simulink model "inclass0912"  (R2022b)
settings: Solver=VariableStepAuto  StartTime=0.0  StopTime=20.0  RelTol=1e-3
settings Model: Creator=sprinkle  LastModifiedBy=sprinkle

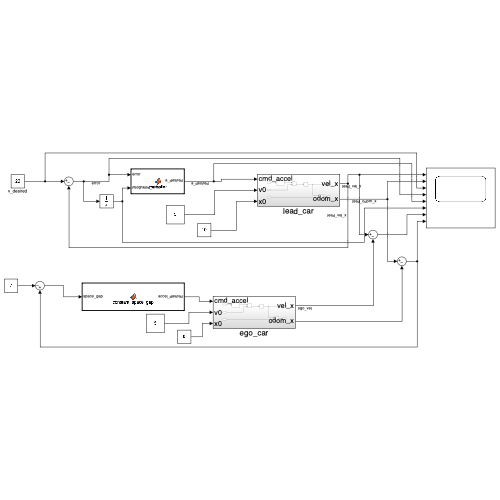
[thumbnail: Simulink's stored preview of the top-level diagram]
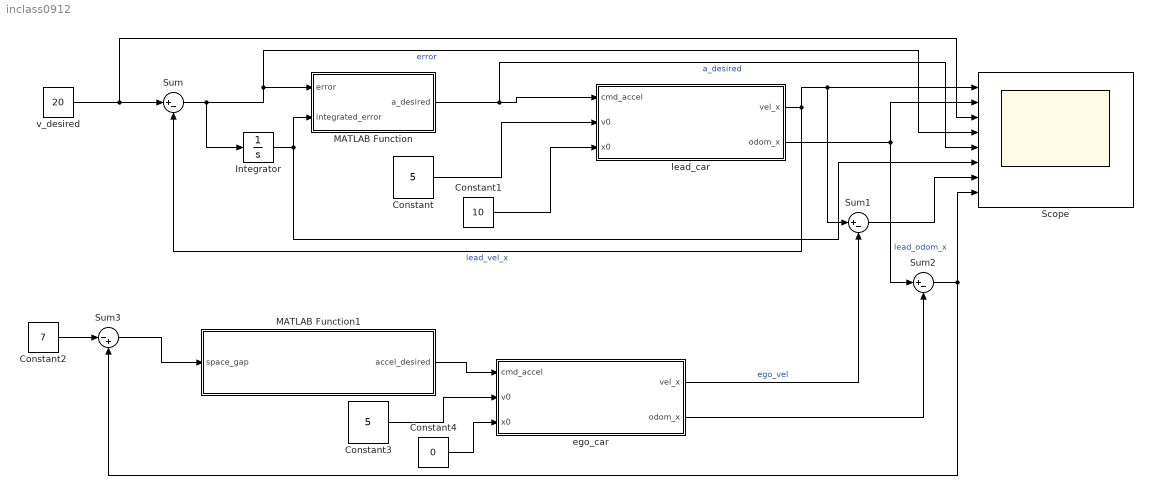
== system inclass0912 ==
  Constant : Constant  Value=5
  Constant1 : Constant  Value=10
  Constant2 : Constant  Value=7
  Constant3 : Constant  Value=5
  Constant4 : Constant  Value=0
  Integrator : Integrator
  MATLAB Function : MATLAB Function  TreatAsAtomicUnit=on
  MATLAB Function1 : MATLAB Function  TreatAsAtomicUnit=on
  Scope : Scope  NumInputPorts=8
  Sum : Sum  Inputs=|+-
  Sum1 : Sum  Inputs=|+-
  Sum2 : Sum  Inputs=|+-
  Sum3 : Sum  Inputs=|-+
  ego_car : Subsystem
  lead_car : Subsystem
  v_desired : Constant  Value=20
  wires:
  Constant/1 -> lead_car/2(v0)
  Constant1/1 -> lead_car/3(x0)
  MATLAB Function/1(a_desired) -> Scope/5, lead_car/1(cmd_accel)  "a_desired"
  lead_car/1(vel_x) -> Sum1/1, Scope/1, Sum/2  "lead_vel_x"
  lead_car/2(odom_x) -> Sum2/1, Scope/2  "lead_odom_x"
  v_desired/1 -> Scope/3, Sum/1
  Sum/1 -> Integrator/1, Scope/4, MATLAB Function/1(error)  "error"
  Integrator/1 -> Scope/6, MATLAB Function/2(integrated_error)
  ego_car/1(vel_x) -> Sum1/2  "ego_vel"
  ego_car/2(odom_x) -> Sum2/2
  Constant2/1 -> Sum3/1
  Sum2/1 -> Scope/8, Sum3/2
  Sum3/1 -> MATLAB Function1/1(space_gap)
  MATLAB Function1/1(accel_desired) -> ego_car/1(cmd_accel)
  Constant3/1 -> ego_car/2(v0)
  Constant4/1 -> ego_car/3(x0)
  Sum1/1 -> Scope/7

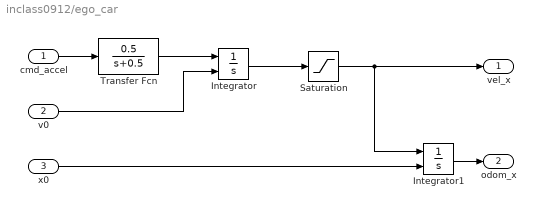
== system inclass0912/ego_car ==
  cmd_accel : Inport
  v0 : Inport  Port=2
  x0 : Inport  Port=3
  Integrator : Integrator  InitialConditionSource=external
  Integrator1 : Integrator  InitialConditionSource=external
  Saturation : Saturate  UpperLimit=80  LowerLimit=0
  Transfer Fcn : TransferFcn  Numerator=[0.5]  Denominator=[1 0.5]
  vel_x : Outport
  odom_x : Outport  Port=2
  wires:
  v0/1 -> Integrator/2
  cmd_accel/1 -> Transfer Fcn/1
  Transfer Fcn/1 -> Integrator/1
  Integrator1/1 -> odom_x/1
  Integrator/1 -> Saturation/1
  x0/1 -> Integrator1/2
  Saturation/1 -> vel_x/1, Integrator1/1

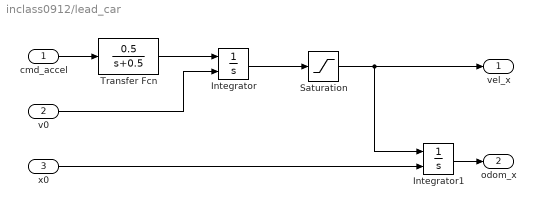
== system inclass0912/lead_car ==
  cmd_accel : Inport
  v0 : Inport  Port=2
  x0 : Inport  Port=3
  Integrator : Integrator  InitialConditionSource=external
  Integrator1 : Integrator  InitialConditionSource=external
  Saturation : Saturate  UpperLimit=80  LowerLimit=0
  Transfer Fcn : TransferFcn  Numerator=[0.5]  Denominator=[1 0.5]
  vel_x : Outport
  odom_x : Outport  Port=2
  wires:
  v0/1 -> Integrator/2
  cmd_accel/1 -> Transfer Fcn/1
  Transfer Fcn/1 -> Integrator/1
  Integrator1/1 -> odom_x/1
  Integrator/1 -> Saturation/1
  x0/1 -> Integrator1/2
  Saturation/1 -> vel_x/1, Integrator1/1

== matlab function inclass0912/MATLAB Function ==
  data: error input; a_desired output; integrated_error input
function a_desired = controller(error,integrated_error)

a_desired = 0.3*error + 0.01*integrated_error;

== matlab function inclass0912/MATLAB Function1 ==
  data: space_gap input; accel_desired output
function accel_desired = constant_space_gap(space_gap)

% tau=0.1;
s_desired=5;
alpha=0.1;

accel_desired = alpha*(space_gap-s_desired);
